simulink model "chap6_3sim"  (Simulink 8.1)
settings: Solver=ode45  StartTime=0.0  StopTime=30  FixedStep=0.001  RelTol=1e-3
settings Model: Creator=ljk  LastModifiedBy=liujk  ExtModeTrigMode=oneshot  ExtModeArmWhenConnect=off
settings DataIOCC: LimitDataPoints=off  SignalLoggingName=sigsOut
settings OptimizationCC: BooleanDataType=off
settings DebuggingCC: SaveWithParameterizedLinksMsg=none  SignalResolutionControl=TryResolveAllWithWarning  SolverPrmCheckMsg=none  MultiTaskDSMMsg=warning  MultiTaskCondExecSysMsg=none  StrictBusMsg=None
settings HardwareCC: TargetUnknown=on
settings RTWCC: IncludeERTFirstTime=on

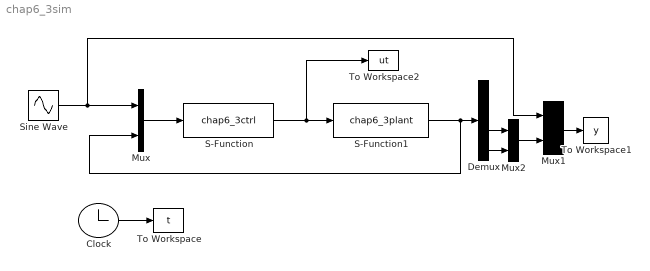
== system chap6_3sim ==
  Clock : Clock
  Demux : Demux
  Mux : Mux  Inputs=2
  Mux1 : Mux  Inputs=2
  Mux2 : Mux  Inputs=2
  S-Function : S-Function  FunctionName=chap6_3ctrl  EnableBusSupport=off
  S-Function1 : S-Function  FunctionName=chap6_3plant  EnableBusSupport=off
  Sine Wave : Sin  SampleTime=0
  To Workspace : ToWorkspace  VariableName=t  SampleTime=-1
  To Workspace1 : ToWorkspace  VariableName=y  SampleTime=-1
  To Workspace2 : ToWorkspace  VariableName=ut  SampleTime=-1
  wires:
  Sine Wave/1 -> Mux1/1, Mux/1
  Mux1/1 -> To Workspace1/1
  S-Function/1 -> S-Function1/1, To Workspace2/1
  S-Function1/1 -> Demux/1, Mux/2
  Mux/1 -> S-Function/1
  Clock/1 -> To Workspace/1
  Mux2/1 -> Mux1/2
  Demux/3 -> Mux2/1
  Demux/4 -> Mux2/2
